simulink model "problema1"  (R2016a)
settings: Solver=FixedStepAuto  StartTime=0.0  StopTime=10.0  FixedStep=0.001  RelTol=1e-3
settings Model: Creator=usuario17  LastModifiedBy=usuario18

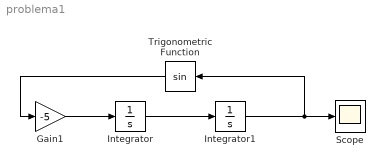
== system problema1 ==
  Gain1 : Gain  Gain=-5
  Integrator : Integrator  InitialCondition=pi/2
  Integrator1 : Integrator  InitialCondition=pi/2
  Scope : Scope
  Trigonometric Function : Trigonometry
  wires:
  Integrator/1 -> Integrator1/1
  Integrator1/1 -> Scope/1, Trigonometric Function/1
  Gain1/1 -> Integrator/1
  Trigonometric Function/1 -> Gain1/1
